simulink model "se_dcdcbuckconverter"  (R2014a)
settings: Solver=ode15s  StartTime=0.0  StopTime=0.005  RelTol=1e-4
StartFcn:
  | tic;
StopFcn:
  | toc;
libraries: fl_lib x13, elec_lib x6, nesl_utility x5
settings Model: Creator=cosorio  LastModifiedBy=cosorio
settings DataIOCC: LimitDataPoints=off  SignalLoggingSaveFormat=ModelDataLogs  SaveOutput=off  SignalLogging=off  SaveTime=off
settings OptimizationCC: ExpressionDepthLimit=2147483647
settings DebuggingCC: UnderspecifiedInitializationDetection=Classic  SolverPrmCheckMsg=none  FcnCallInpInsideContextMsg=UseLocalSettings  StateNameClashWarn=warning
settings GRTTargetCC: CombineOutputUpdateFcns=off  GRTInterface=on

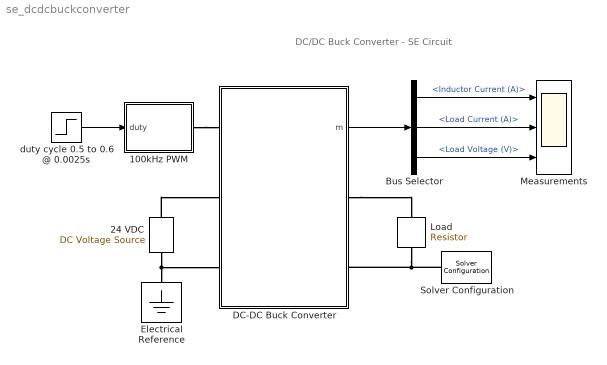
== system se_dcdcbuckconverter ==
  note: DC/DC Buck Converter - SE Circuit
  100kHz PWM : Subsystem
  24 VDC : fl_lib/Electrical/Electrical Sources/DC Voltage Source  v0=24 V
  Bus Selector : BusSelector  OutputSignals=Inductor Current (A),Load Current (A),Load Voltage (V)
  DC-DC Buck Converter : Subsystem
  Electrical Reference : fl_lib/Electrical/Electrical Elements/Electrical Reference
  Load : fl_lib/Electrical/Electrical Elements/Resistor  R=2.4 Ohm  i_specify=off  i_priority=High  i=5 A  v_specify=off  v_priority=High  v=0 V
  Measurements : Scope  NumInputPorts=3
      settings: YMin=0~0~0  YMax=10~10~20  SaveName=BuckSE
  Solver Configuration : nesl_utility/Solver Configuration  PhysicalDomain=network_engine_domain  SubClassName=solver  LeftPortType=input  RightPortType=generic  Accelerate=off  Tones=[]  Harmonics=[]  SimulateNoise=off  Profile=off  UseLocalSampling=off  EnableSwitchedLinearOptims=on  FrequencyDomain=off  UseCCode=off  RelTol=0.001  AbsTol=1e-06  MinStep=1e-09  ToWorkspace=off  DoDC=off  ResidualTolerance=1e-9  UseLocalSolver=off  LocalSolverChoice=NE_BACKWARD_EULER_ADVANCER  LocalSolverSampleTime=1e-7  DoFixedCost=off  MaxNonlinIter=4  MaxModeIter=2  LinearAlgebra=Sparse  DelaysMemoryBudget=1024  AutomaticFiltering=on  FilteringTimeConstant=0.001
  duty cycle 0.5 to 0.6 @ 0.0025s : Step  Time=0.0025  Before=50  After=60  SampleTime=0
  wires:
  duty cycle 0.5 to 0.6 @ 0.0025s/1 -> 100kHz PWM/1(duty)
  DC-DC Buck Converter/1(m) -> Bus Selector/1
  Bus Selector/1 -> Measurements/1  "<Inductor Current (A)>"
  Bus Selector/3 -> Measurements/3  "<Load Voltage (V)>"
  Bus Selector/2 -> Measurements/2  "<Load Current (A)>"
  connections:
  24 VDC/RConn1 -- Electrical Reference/LConn1 -- DC-DC Buck Converter/LConn3
  24 VDC/LConn1 -- DC-DC Buck Converter/LConn2
  100kHz PWM/RConn1 -- DC-DC Buck Converter/LConn1
  DC-DC Buck Converter/RConn1 -- Load/LConn1
  Solver Configuration/RConn1 -- Load/RConn1 -- DC-DC Buck Converter/RConn2

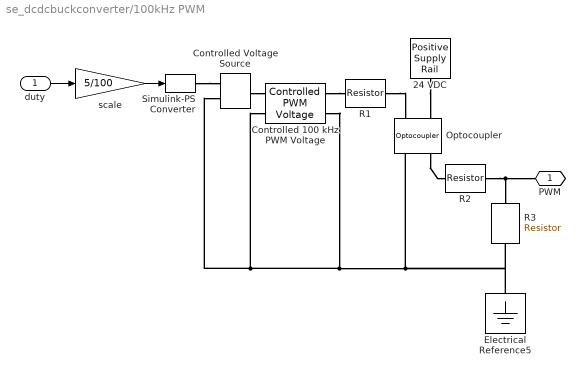
== system se_dcdcbuckconverter/100kHz PWM ==
  duty : Inport
  24 VDC : elec_lib/Sources/Positive Supply Rail  v0=24 V
  Controlled 100 kHz PWM Voltage : elec_lib/Actuators & Drivers/Drivers/Controlled PWM Voltage  F=1e05 Hz  TD=0 s  pulse_width_offset=0 s  Vmin=0 V  Vmax=5 V  Vm=5 V  pwm_or_av=1  event_type=1  sample_time=1e-6 s
  Controlled Voltage Source : fl_lib/Electrical/Electrical Sources/Controlled Voltage Source
  Electrical Reference5 : fl_lib/Electrical/Electrical Elements/Electrical Reference
  Optocoupler : elec_lib/Semiconductor Devices/Optocoupler  CTR=0.35  prmExp=1  I12=[0.001 0.015] A  V12=[0.9 1.05] V  RS=0 Ohm  IS=1e-10 A  Tmeas=298.15 K  ec=2  C_param=1  CJ0=50 pF  VJ=1 V  Mgrad=0.5  Vvec="[  0.1 10 100 ] V"  Cvec="[  3.5 1 0.4 ] pF"  FC=0.5  T_param=1  IS_T2=1.8e-8 A  I1_T2=0.029 A  V1_T2=1.05 V  Tmeas2=125 C  EG_param=1  EG=1.11 eV  XTI_param=1  XTI=3  Tdevice=25 C  Rth=[ 0 10 ] K/W  thermal_mass_parameterization=1  thermal_mass=[ 0 1 ] J/K  thermal_time_constant=[ 0 10 ] s  thermal_mass_initial_temperatures=[ 25 25 ] C
  R1 : fl_lib/Electrical/Electrical Elements/Resistor  R=1100 Ohm  i_specify=off  i_priority=High  i=0 A  v_specify=off  v_priority=High  v=0 V
  R2 : fl_lib/Electrical/Electrical Elements/Resistor  R=10e3 Ohm  i_specify=off  i_priority=High  i=0 A  v_specify=off  v_priority=High  v=0 V
  R3 : fl_lib/Electrical/Electrical Elements/Resistor  R=22.5e3 Ohm  i_specify=off  i_priority=High  i=0 A  v_specify=off  v_priority=High  v=0 V
  Simulink-PS Converter : nesl_utility/Simulink-PS Converter  PhysicalDomain=network_engine_domain  SubClassName=ps_input  LeftPortType=input  RightPortType=output  PseudoPeriodic=off  Frequencies=[]  NoiseDistribution=none  NoiseParameters=[]  Unit=V  AffineConversion=off  InputFiltering=off  SimscapeFilterOrder=1  InputFilterTimeConstant=.001  UdotUserProvided=0
  scale : Gain  Gain=5/100
  PWM : PMIOPort  Port=1  Side=Right
  wires:
  duty/1 -> scale/1
  scale/1 -> Simulink-PS Converter/1
  connections:
  Controlled Voltage Source/LConn1 -- Controlled 100 kHz PWM Voltage/LConn1
  Simulink-PS Converter/RConn1 -- Controlled Voltage Source/RConn1
  24 VDC/RConn1 -- Optocoupler/LConn2
  Controlled 100 kHz PWM Voltage/RConn1 -- R1/RConn1
  Optocoupler/RConn2 -- R2/LConn1
  R2/RConn1 -- R3/LConn1 -- PWM/RConn1
  Controlled 100 kHz PWM Voltage/RConn2 -- Controlled 100 kHz PWM Voltage/LConn2 -- Controlled Voltage Source/RConn2 -- Electrical Reference5/LConn1 -- R3/RConn1 -- Optocoupler/RConn1
  R1/LConn1 -- Optocoupler/LConn1

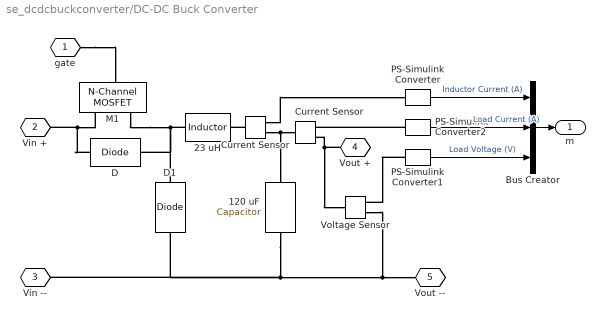
== system se_dcdcbuckconverter/DC-DC Buck Converter ==
  120 uF : fl_lib/Electrical/Electrical Elements/Capacitor  c=120e-06 F  r=0.25 Ohm  g=0 1/Ohm  i_specify=off  i_priority=High  i=0 A  v_specify=on  v_priority=High  v=0 V  vc_specify=off  vc_priority=High  vc=12 V
  23 uH : fl_lib/Electrical/Electrical Elements/Inductor  l=23e-06 H  r=0.05 Ohm  g=1e-09 1/Ohm  i_specify=off  i_priority=High  i=0 A  v_specify=off  v_priority=High  v=0 V  i_L_specify=off  i_L_priority=High  i_L=5 A
  Bus Creator : BusCreator  Inputs=3
  Current Sensor : fl_lib/Electrical/Electrical Sensors/Current Sensor
  "Current Sensor " : fl_lib/Electrical/Electrical Sensors/Current Sensor
  D : elec_lib/Semiconductor Devices/Diode  ModelType=3  Vf=0.7 V  Ron=0.01 Ohm  Goff=1e-08 S  Rz=0.3 Ohm  Vz=50 V  C_PWL=5 pF  prmExp=1  I12=[0.07 1.5 ] A  V12=[0.7 0.8 ] V  I1=0.0137 A  V1=0.6 V  RS=0.01 Ohm  IS=1e-14 A  Tmeas=25 C  ec=1  BV=Inf V  C_param=1  CJ0=5 pF  VJ=1 V  Mgrad=0.5  Vvec="[  0.1 10 100 ] V"  Cvec="[  3.5 1 0.4 ] pF"  FC=0.5  Q_param=1  Irrm=-7.15 A  iF=4 A  didt=-750 A/us  trr=115 ns  TT=50 ns  tau=100 ns  T_param=1  IS_T2=1.25e-7 A  I1_T2=0.245 A  V1_T2=0.5 V  Tmeas2=125 C  EG_param=1  EG=1.11 eV  XTI_param=1  XTI=3  dBVdT=0 V/K  Tdevice=25 C  Rth=[ 0 10 ] K/W  thermal_mass_parameterization=1  thermal_mass=[ 0 1 ] J/K  thermal_time_constant=[ 0 10 ] s  thermal_mass_initial_temperatures=[ 25 25 ] C
  D1 : elec_lib/Semiconductor Devices/Diode  ModelType=3  Vf=0.7 V  Ron=0.01 Ohm  Goff=1e-08 S  Rz=0.3 Ohm  Vz=50 V  C_PWL=5 pF  prmExp=1  I12=[0.07 1.5 ] A  V12=[0.7 0.8 ] V  I1=0.0137 A  V1=0.6 V  RS=0.01 Ohm  IS=1e-14 A  Tmeas=25 C  ec=1  BV=Inf V  C_param=1  CJ0=5 pF  VJ=1 V  Mgrad=0.5  Vvec="[  0.1 10 100 ] V"  Cvec="[  3.5 1 0.4 ] pF"  FC=0.5  Q_param=1  Irrm=-7.15 A  iF=4 A  didt=-750 A/us  trr=115 ns  TT=50 ns  tau=100 ns  T_param=1  IS_T2=1.25e-7 A  I1_T2=0.245 A  V1_T2=0.5 V  Tmeas2=125 C  EG_param=1  EG=1.11 eV  XTI_param=1  XTI=3  dBVdT=0 V/K  Tdevice=25 C  Rth=[ 0 10 ] K/W  thermal_mass_parameterization=1  thermal_mass=[ 0 1 ] J/K  thermal_time_constant=[ 0 10 ] s  thermal_mass_initial_temperatures=[ 25 25 ] C
  M1 : elec_lib/Semiconductor Devices/N-Channel MOSFET  parameterization=1  prmDatasheet=1  prmEquCoeff=1  Beta=5 A/V^2  Rds=0.0025 Ohm  Id=6 A  Vgs=20 V  Vth=2.5 V  lam=0 1/V  Tmeas=25 C  RS=0.001 Ohm  RD=0.001 Ohm  C_param=1  C_GS=270 pF  C_GD=80 pF  C_iss=350 pF  C_rss=80 pF  C_oss=0 pF  charge_linearity_param=1  C_OX=200 pF  V_C_OX=-0.5 V  dVth_dT=-6 mV/K  Rds_T2=0.037 Ohm  Tmeas2=125 C  BEXDatasheet=-1.5  BEXEquCoeff=-1.5  TdeviceDatasheet=25 C  TdeviceEquCoeff=25 C  Rth=[ 0 10 ] K/W  thermal_mass_parameterization=1  thermal_mass=[ 0 1 ] J/K  thermal_time_constant=[ 0 10 ] s  thermal_mass_initial_temperatures=[ 25 25 ] C
  PS-Simulink Converter : nesl_utility/PS-Simulink Converter  PhysicalDomain=network_engine_domain  SubClassName=ps_output  LeftPortType=input  RightPortType=output  PseudoPeriodic=off  Frequencies=[]  Unit=A  AffineConversion=off
  PS-Simulink Converter1 : nesl_utility/PS-Simulink Converter  PhysicalDomain=network_engine_domain  SubClassName=ps_output  LeftPortType=input  RightPortType=output  PseudoPeriodic=off  Frequencies=[]  Unit=V  AffineConversion=off
  PS-Simulink Converter2 : nesl_utility/PS-Simulink Converter  PhysicalDomain=network_engine_domain  SubClassName=ps_output  LeftPortType=input  RightPortType=output  PseudoPeriodic=off  Frequencies=[]  Unit=A  AffineConversion=off
  Voltage Sensor : fl_lib/Electrical/Electrical Sensors/Voltage Sensor
  gate : PMIOPort  Tag=PMCPort  Port=1  Side=Left
  Vin + : PMIOPort  Tag=PMCPort  Port=2  Side=Left
  Vin -- : PMIOPort  Tag=PMCPort  Port=3  Side=Left
  Vout + : PMIOPort  Tag=PMCPort  Port=4  Side=Right
  Vout -- : PMIOPort  Tag=PMCPort  Port=5  Side=Right
  m : Outport
  wires:
  PS-Simulink Converter/1 -> Bus Creator/1  "Inductor Current (A)"
  Bus Creator/1 -> m/1
  PS-Simulink Converter1/1 -> Bus Creator/3  "Load Voltage (V)"
  PS-Simulink Converter2/1 -> Bus Creator/2  "Load Current (A)"
  connections:
  Current Sensor/RConn2 -- "Current Sensor "/LConn1 -- 120 uF/LConn1
  23 uH/LConn1 -- D/LConn1 -- M1/RConn2 -- D1/RConn1
  Current Sensor/RConn1 -- PS-Simulink Converter/LConn1
  D/RConn1 -- Vin +/RConn1 -- M1/RConn1
  gate/RConn1 -- M1/LConn1
  PS-Simulink Converter1/LConn1 -- Voltage Sensor/RConn1
  D1/LConn1 -- Vin --/RConn1 -- 120 uF/RConn1 -- Voltage Sensor/RConn2 -- Vout --/RConn1
  Current Sensor/LConn1 -- 23 uH/RConn1
  Vout +/RConn1 -- "Current Sensor "/RConn2 -- Voltage Sensor/LConn1
  PS-Simulink Converter2/LConn1 -- "Current Sensor "/RConn1
